simulink model "Simulink"  (R2022b)
settings: Solver=VariableStepAuto  StartTime=0.0  StopTime=00.0  RelTol=1e-3
settings Model: Creator=ECAD-30  LastModifiedBy=ECAD-30

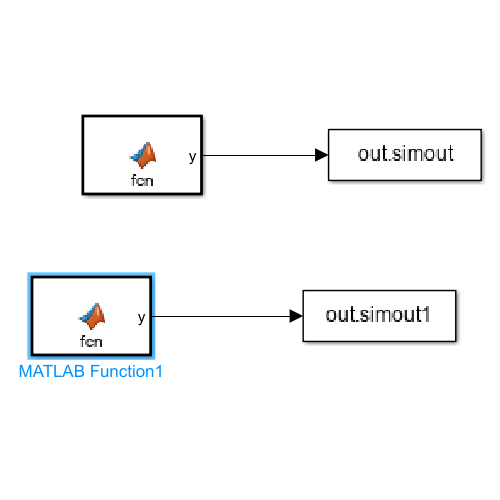
[thumbnail: Simulink's stored preview of the top-level diagram]
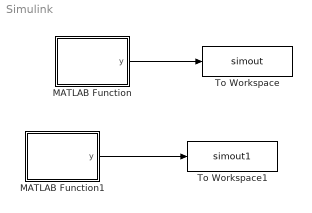
== system Simulink ==
  MATLAB Function : MATLAB Function  TreatAsAtomicUnit=on
  MATLAB Function1 : MATLAB Function  TreatAsAtomicUnit=on
  To Workspace : ToWorkspace  VariableName=simout  SampleTime=.1
      settings: Save2DSignal=2-D array (concatenate along first dimension)
  To Workspace1 : ToWorkspace  VariableName=simout1  SampleTime=.1
      settings: Save2DSignal=2-D array (concatenate along first dimension)
  wires:
  MATLAB Function/1(y) -> To Workspace/1
  MATLAB Function1/1(y) -> To Workspace1/1

== matlab function Simulink/MATLAB Function ==
  data: y output
function y = fcn()

A = 0.5;
f = 3000;
Fs = 1e5;
%n = 0:1:4*(f/fs);
t = linspace(0,4/f,1000);

x = A * cos(2*pi*(f)*t);

y = x;

== matlab function Simulink/MATLAB Function1 ==
  data: y output
function y = fcn()

Fs = 12000;
A = 0.5;
f = 3000;
N=4;
for i=1:5
   n1 = 0:1:4*(Fs/f);
   x1 = A*cos(2*pi*n1*(f/Fs));
   
   

end
y = x1;
